simulink model "pendulosimulink"  (R2019b)
settings: Solver=ode15s  StartTime=0.0  StopTime=50  FixedStep=0.1  RelTol=0.001  AbsTol=0.001
settings Model: Creator=Fer  LastModifiedBy=Fer
settings SolverCC: AutoScaleAbsTol=off

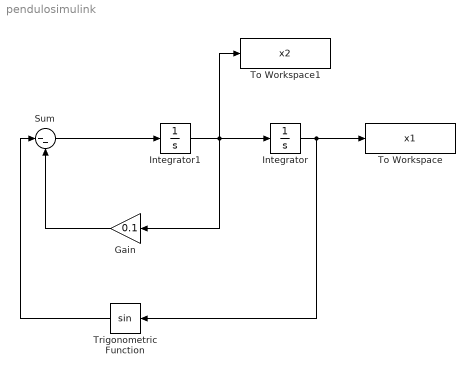
== system pendulosimulink ==
  Gain : Gain  Gain=0.1
  Integrator : Integrator  InitialCondition=1
  Integrator1 : Integrator
  Sum : Sum  Inputs=|--
  To Workspace : ToWorkspace  VariableName=x1  SaveFormat=Structure With Time  SampleTime=-1
      settings: Decimation=10
  To Workspace1 : ToWorkspace  VariableName=x2  SaveFormat=Structure With Time  SampleTime=-1
      settings: Decimation=10
  Trigonometric Function : Trigonometry
  wires:
  Sum/1 -> Integrator1/1
  Integrator1/1 -> To Workspace1/1, Gain/1, Integrator/1
  Trigonometric Function/1 -> Sum/1
  Gain/1 -> Sum/2
  Integrator/1 -> To Workspace/1, Trigonometric Function/1
